simulink model "verify_StorageTnodesEN12977hx_mdl"  (Simulink 8.2)
settings: Solver=ode45  StartTime=0.0  StopTime=24*3600  MaxStep=900  RelTol=1e-3
libraries: carnot x12
settings Model: Creator=drhf  LastModifiedBy=drhf
settings DataIOCC: LimitDataPoints=off

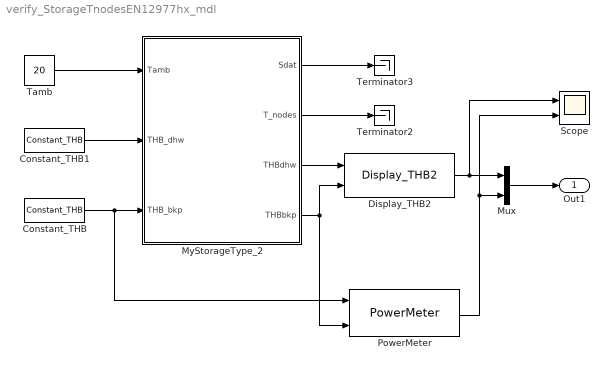
== system verify_StorageTnodesEN12977hx_mdl ==
  Constant_THB : carnot/Source/Simple/Constant_THB  t=90  mdot=200/3600  p=1e5  mID=No Pressure Drop  fluid=Water (Constant 20°C)  mix=0  dia=0.02  hgt=0
  Constant_THB1 : carnot/Source/Simple/Constant_THB  t=20  mdot=600/3600  p=1e5  mID=No Pressure Drop  fluid=Water (Constant 20°C)  mix=0  dia=0.02  hgt=0
  Display_THB2 : carnot/Outputs/Display_THB2  t=on  m=off  p=off  id=off  mix=off  d=off
  Mux : Mux  Inputs=2
  MyStorageType_2 : Subsystem  mask(Multiport Storage){uloss=0, ubot=0, utop=0, cond=0, t0=30, volume=0.3, dia=0.5, pos=standing cylinder, nconnect=2, nodes=100, mpoints=100}
      mask prompts: uloss "Heat loss coefficient cylinder wall in W/(m²K)"; ubot "Heat loss coefficient bottom in W/(m²K)"; utop "Heat loss coefficient top cover in W/(m²K)"; cond "Effective vertical conductivity in W/(m*K)"; t0 "Initial temperature (vector or scalar) in °C"; volume "Volume in m³"; dia "Diameter in m"; pos "Position"; nconnect "Number of connections"; nodes "Number of nodes"; mpoints "Number of measurement points"
      mask help:
      | The volmue of the cylindrical storage is divided in a number "nodes" of horizontal slices (1xN-node model). For each node the energy balance equation is solved.
      | Look under mask to set the ports types and properties.
      mask init:
      | [standing, dh, height, mpts, tini] ...
      |     = CarnotCallbacks_StorageTypeN(pos, volume, dia, nodes, mpoints, t0);
      mask Help: eval('man(''storage_multiport'')')
      mask TypeOptions pos: lying cylinder | standing cylinder
      mask Display: plot(10,20,80,100,[36,36,40,50,54,54,50,40,36],[90,50,45,45,50,90,93,93,90],[36,51,44,51,36],[50,50,55,60,60])
  PowerMeter : carnot/Control/PowerMeter
  Scope : Scope  NumInputPorts=2
      settings: YMin=-5~-5  YMax=5~5
  Tamb : Constant  Value=20
  Terminator2 : Terminator
  Terminator3 : Terminator
  Out1 : Outport
  wires:
  Tamb/1 -> MyStorageType_2/1(Tamb)
  MyStorageType_2/1(Sdat) -> Terminator3/1
  MyStorageType_2/2(T_nodes) -> Terminator2/1
  MyStorageType_2/3(THBdhw) -> Display_THB2/1
  MyStorageType_2/4(THBbkp) -> Display_THB2/2, PowerMeter/2
  Display_THB2/1 -> Mux/1, Scope/1
  Mux/1 -> Out1/1
  Constant_THB1/1 -> MyStorageType_2/2(THB_dhw)
  Constant_THB/1 -> MyStorageType_2/3(THB_bkp), PowerMeter/1
  PowerMeter/1 -> Mux/2, Scope/2

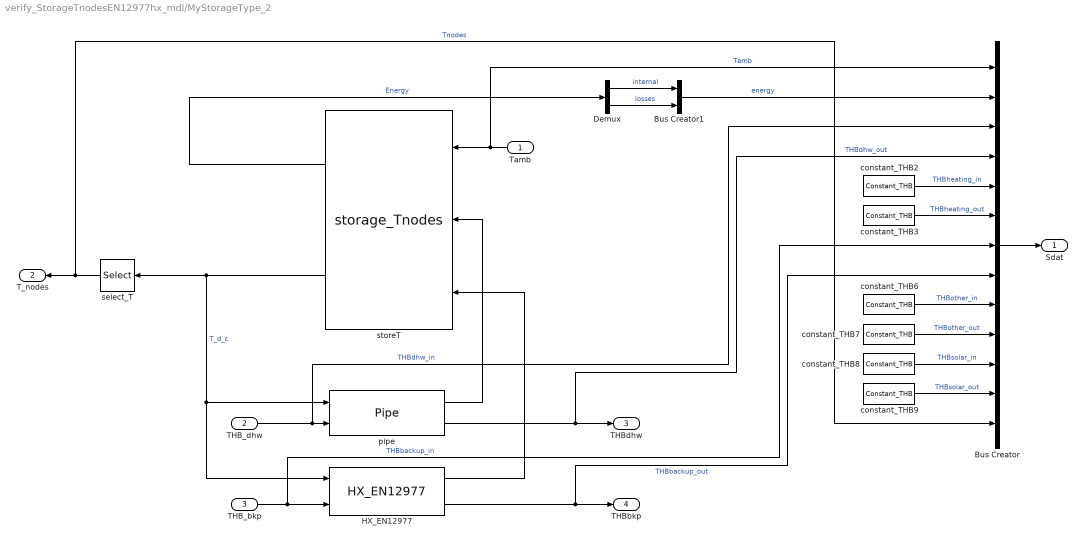
== system verify_StorageTnodesEN12977hx_mdl/MyStorageType_2 ==
  Tamb : Inport
  THB_dhw : Inport  Port=2
  THB_bkp : Inport  Port=3
  Bus Creator : BusCreator  Inputs=13
  Bus Creator1 : BusCreator  Inputs=2
  Demux : Demux  Outputs=2
  HX_EN12977 : carnot/Storage/Thermal/Storage_Ports/HX_EN12977  h_in=1  h_out=0  ua0=1667  uam=0  uat=0  dplin=100  dpqua=100  nodes=nodes  hgt=height  dia=dia
  constant_THB{2..3,6..9} (6 alike) : carnot/Source/Simple/Constant_THB  t=20  mdot=0  p=1e5  mID=No Pressure Drop  fluid=Water  mix=0  dia=0.02  hgt=0
  pipe : carnot/Storage/Thermal/Storage_Ports/Pipe  h_in=0  h_out=1  nodes=nodes  hgt=height  dia=dia  dplin=10  dpqua=10
  select_T : Selector  InputPortWidth=nodes  IndexOptions=Index vector (dialog)  Indices=mpts  OutputSizes=1
  storeT : S-Function  FunctionName=storage_Tnodes  Parameters=dia, volume, standing, uloss , ubot, utop, cond, tini, nodes, nconnect  EnableBusSupport=off
  Sdat : Outport
  T_nodes : Outport  Port=2
  THBdhw : Outport  Port=3
  THBbkp : Outport  Port=4
  wires:
  Tamb/1 -> storeT/1, Bus Creator/1  "Tamb"
  THB_dhw/1 -> Bus Creator/3, pipe/2  "THBdhw_in"
  pipe/2 -> Bus Creator/4, THBdhw/1  "THBdhw_out"
  pipe/1 -> storeT/2
  select_T/1 -> T_nodes/1, Bus Creator/13  "Tnodes"
  storeT/1 -> Demux/1  "Energy"
  storeT/2 -> select_T/1, pipe/1, HX_EN12977/1  "T_d_c"
  Bus Creator/1 -> Sdat/1
  constant_THB9/1 -> Bus Creator/12  "THBsolar_out"
  constant_THB8/1 -> Bus Creator/11  "THBsolar_in"
  constant_THB7/1 -> Bus Creator/10  "THBother_out"
  constant_THB6/1 -> Bus Creator/9  "THBother_in"
  constant_THB2/1 -> Bus Creator/5  "THBheating_in"
  constant_THB3/1 -> Bus Creator/6  "THBheating_out"
  THB_bkp/1 -> Bus Creator/7, HX_EN12977/2  "THBbackup_in"
  HX_EN12977/2 -> Bus Creator/8, THBbkp/1  "THBbackup_out"
  HX_EN12977/1 -> storeT/3
  Demux/1 -> Bus Creator1/1  "internal"
  Demux/2 -> Bus Creator1/2  "losses"
  Bus Creator1/1 -> Bus Creator/2  "energy"
